simulink model "Contin"  (R2014b)
settings: Solver=ode45  SolverMode=SingleTasking  StartTime=0.0  StopTime=10.0  MaxStep=.001  RelTol=1e-3  AbsTol=1e-6
undefined symbols (not defined in the file): B, fd, Ka, Kd, Ki, Kp, M, taua, v0, vref
settings Model: ExtModeAutoUpdateStatusClock=off  Creator=mcb  LastModifiedBy=mcberg
settings DataIOCC: LimitDataPoints=off  SignalLoggingSaveFormat=ModelDataLogs  SaveOutput=off  SaveTime=off  TimeSaveName=time  SignalLoggingName=sigsOut
settings OptimizationCC: BooleanDataType=off
settings DebuggingCC: SaveWithParameterizedLinksMsg=none  UnderspecifiedInitializationDetection=Classic  MergeDetectMultiDrivingBlocksExec=none  SignalResolutionControl=TryResolveAllWithWarning  SolverPrmCheckMsg=none  MultiTaskDSMMsg=warning  MultiTaskCondExecSysMsg=none  FcnCallInpInsideContextMsg=EnableAllAsWarning
settings HardwareCC: TargetUnknown=on
settings RTWCC: TemplateMakefile=grt_vc.tmf  IncludeERTFirstTime=on
settings GRTTargetCC: CombineOutputUpdateFcns=off  GRTInterface=on

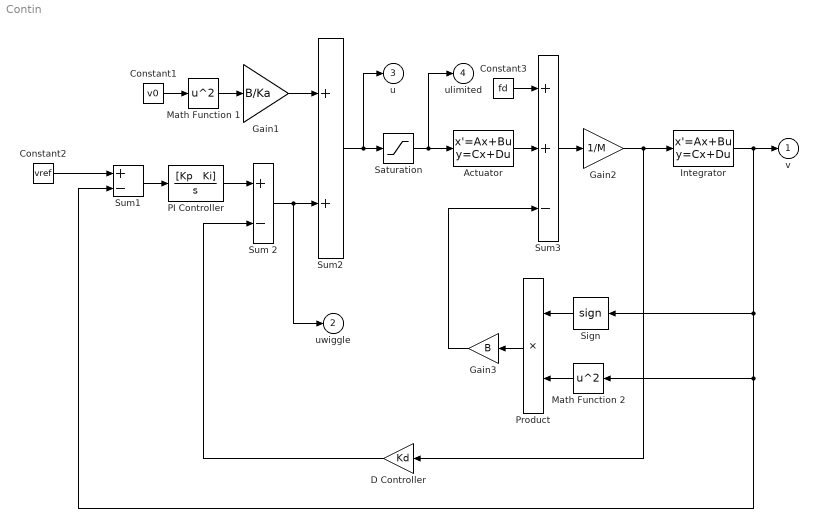
== system Contin ==
  Actuator : StateSpace  A=-1/taua  B=Ka/taua  D=0  X0=B*v0^2
  Constant1 : Constant  Value=v0
  Constant2 : Constant  Value=vref
  Constant3 : Constant  Value=fd
  D Controller : Gain  Gain=Kd  SaturateOnIntegerOverflow=on  OutDataTypeStr=Inherit: Same as input  ParamDataTypeStr=Inherit: Same as input
  Gain1 : Gain  Gain=B/Ka  SaturateOnIntegerOverflow=on  OutDataTypeStr=Inherit: Same as input  ParamDataTypeStr=Inherit: Same as input
  Gain2 : Gain  Gain=1/M  SaturateOnIntegerOverflow=on  OutDataTypeStr=Inherit: Same as input  ParamDataTypeStr=Inherit: Same as input
  Gain3 : Gain  Gain=B  SaturateOnIntegerOverflow=on  OutDataTypeStr=Inherit: Same as input  ParamDataTypeStr=Inherit: Same as input
  Integrator : StateSpace  A=0  D=0  X0=v0
  Math Function 1 : Math  Operator=square  SaturateOnIntegerOverflow=on
  Math Function 2 : Math  Operator=square  SaturateOnIntegerOverflow=on
  PI Controller : TransferFcn  Numerator="[Kp   Ki]"  Denominator="[1   0]"
  Product : Product  SaturateOnIntegerOverflow=on  InputSameDT=on  OutDataTypeStr=Inherit: Same as first input
  Saturation : Saturate  UpperLimit=1  LowerLimit=0
  Sign : Signum
  Sum 2 : Sum  Inputs=+-  SaturateOnIntegerOverflow=on  InputSameDT=on  OutDataTypeStr=Inherit: Same as first input
  Sum1 : Sum  Inputs=+-  SaturateOnIntegerOverflow=on  InputSameDT=on  OutDataTypeStr=Inherit: Same as first input
  Sum2 : Sum  SaturateOnIntegerOverflow=on  InputSameDT=on  OutDataTypeStr=Inherit: Same as first input
  Sum3 : Sum  Inputs=++-  SaturateOnIntegerOverflow=on  InputSameDT=on  OutDataTypeStr=Inherit: Same as first input
  v : Outport  InitialOutput=0
  uwiggle : Outport  Port=2  InitialOutput=0
  u : Outport  Port=3  InitialOutput=0
  ulimited : Outport  Port=4  InitialOutput=0
  wires:
  Constant2/1 -> Sum1/1
  Sum1/1 -> PI Controller/1
  Sign/1 -> Product/1
  Math Function 2/1 -> Product/2
  Product/1 -> Gain3/1
  Gain3/1 -> Sum3/3
  Sum3/1 -> Gain2/1
  Sum2/1 -> Saturation/1, u/1
  Actuator/1 -> Sum3/2
  Saturation/1 -> Actuator/1, ulimited/1
  PI Controller/1 -> Sum 2/1
  Gain1/1 -> Sum2/1
  Sum 2/1 -> Sum2/2, uwiggle/1
  Integrator/1 -> Math Function 2/1, Sum1/2, Sign/1, v/1
  D Controller/1 -> Sum 2/2
  Gain2/1 -> Integrator/1, D Controller/1
  Math Function 1/1 -> Gain1/1
  Constant1/1 -> Math Function 1/1
  Constant3/1 -> Sum3/1
